simulink model "PID_controler"  (R2025b)
settings: Solver=VariableStepAuto  StartTime=0.0  StopTime=t(end)  RelTol=1e-3
values from neighbouring files (symbols this model uses):
  k = 18    [PartOne2_0.m]
  KD = 0.63    [PartOne2_0.m]
  KI = 85    [PartOne2_0.m]
  TaS = 1/10000    (= 0.0001)    [PartOne2_0.m]
  tdelay = 0    [PartOne2_0.m]
libraries: cstblocks x1
settings Model: Creator=Jorben  LastModifiedBy=Jorben

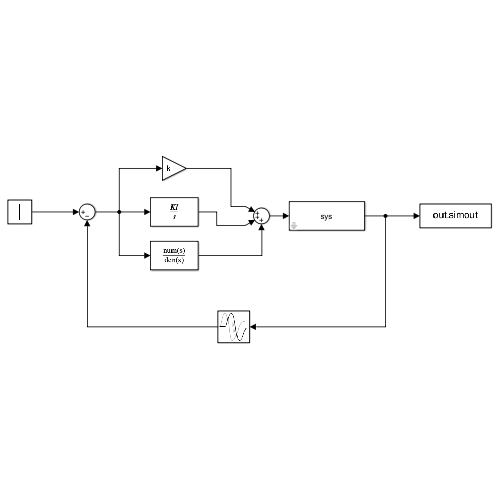
[thumbnail: Simulink's stored preview of the top-level diagram]
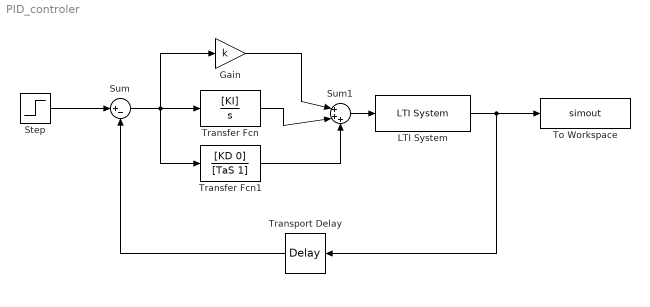
== system PID_controler ==
  Gain : Gain  Gain=k
  LTI System : cstblocks/LTI System  sys=sys  IC=[]  PadeOrder=0
  Step : Step  Time=0.1  SampleTime=t(2) - t(1)
  Sum : Sum  Inputs=|+-
  Sum1 : Sum  Inputs=|+++
  To Workspace : ToWorkspace  VariableName=simout  SampleTime=t(2) - t(1)
  Transfer Fcn : TransferFcn  Numerator=[KI]  Denominator=[1 0]
  Transfer Fcn1 : TransferFcn  Numerator=[KD 0]  Denominator=[TaS 1]
  Transport Delay : TransportDelay  DelayTime=tdelay
  wires:
  Sum/1 -> Transfer Fcn1/1, Transfer Fcn/1, Gain/1
  Gain/1 -> Sum1/1
  Transfer Fcn/1 -> Sum1/2
  Transfer Fcn1/1 -> Sum1/3
  Step/1 -> Sum/1
  Sum1/1 -> LTI System/1
  LTI System/1 -> Transport Delay/1, To Workspace/1
  Transport Delay/1 -> Sum/2
